simulink model "T5"  (R2024a)
settings: Solver=VariableStepAuto  StartTime=0.0  StopTime=40.0  RelTol=1e-3
settings Model: NumberOfSteps=2  Creator=PMYLS  LastModifiedBy=PMYLS

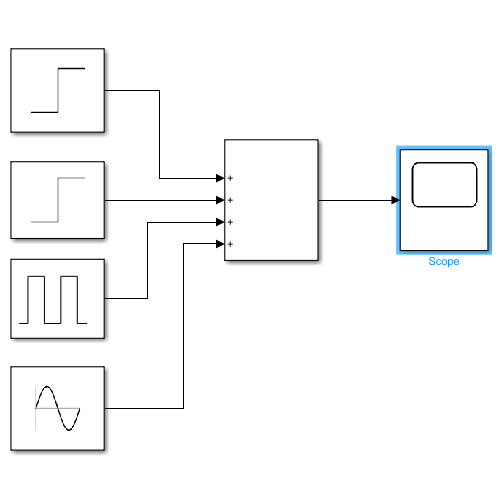
[thumbnail: Simulink's stored preview of the top-level diagram]
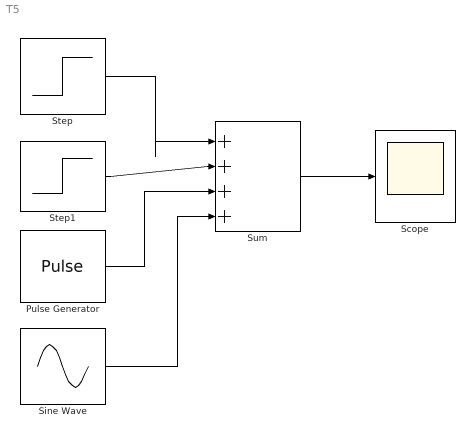
== system T5 ==
  Pulse Generator : DiscretePulseGenerator  PulseType=Time based  Period=10  PulseWidth=50
  Scope : Scope
  Sine Wave : Sin  Frequency=2*pi  SampleTime=0
  Step : Step  SampleTime=0
  Step1 : Step  Time=5  After=2  SampleTime=0
  Sum : Sum  Inputs=|++++
  wires:
  Step/1 -> Sum/1
  Step1/1 -> Sum/2
  Pulse Generator/1 -> Sum/3
  Sine Wave/1 -> Sum/4
  Sum/1 -> Scope/1
